simulink model "ControlSingleV1_3"  (R2015b)
settings: Solver=ode1  StartTime=0.0  StopTime=inf  FixedStep=0.001  RelTol=1e-3
libraries: simulink x1
settings Model: ExtModeTrigDuration=10000  Creator=ale  LastModifiedBy=Le
settings SolverCC: PositivePriorityOrder=on
settings RTWCC: SystemTargetFile=quarc_linux_duovero.tlc  TemplateMakefile=quarc_linux_duovero_tmf  Description=QUARC Linux DuoVero Target (QBall 2, QBot 2)
settings STFCustomTargetCC: TargetLibSuffix=.a  TargetPreCompLibLocation=C:\PROGRA~3\QUARC\lib\2015b\LINUX_~1\release  GeneratePreprocessorConditionals=Use local settings  CPPClassGenCompliant=off  SystemTargetFile=quarc_linux_duovero.tlc
settings GRTTargetCC: TargetLibSuffix=.a  TargetPreCompLibLocation=C:\PROGRA~3\QUARC\lib\2015b\LINUX_~1\release  ParMdlRefBuildCompliant=off  CompOptLevelCompliant=off  CombineOutputUpdateFcns=off  MatFileLogging=off  CPPClassGenCompliant=off  GRTInterface=on  UseToolchainInfoCompliant=off  ExtMode=on  ExtModeMexFile=quarc_comm  ExtModeMexArgs='-w -d /tmp -uri %u'

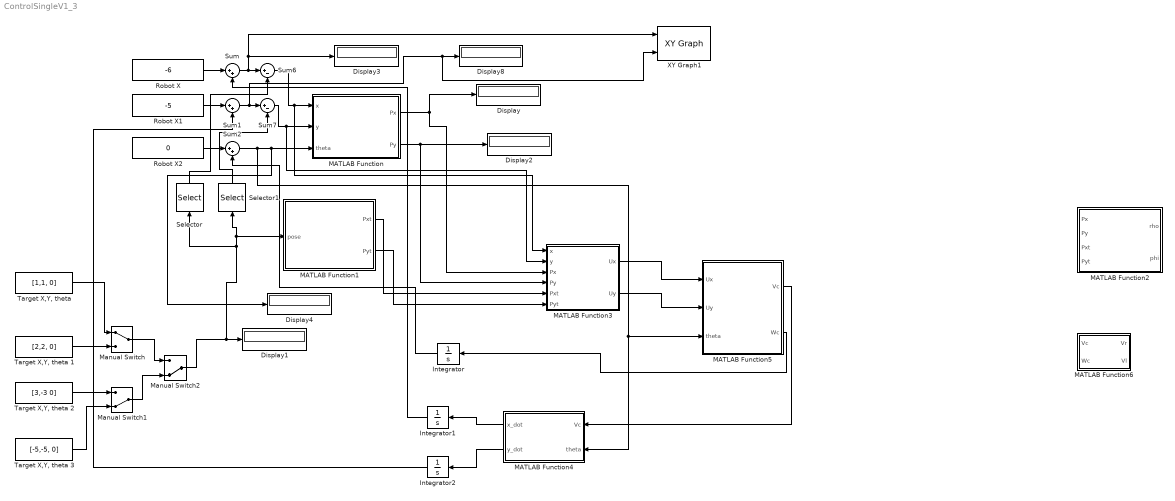
== system ControlSingleV1_3 ==
  Display{,1..4,8} (6 alike) : Display
  Integrator : Integrator
  Integrator1 : Integrator
  Integrator2 : Integrator
  MATLAB Function : MATLAB Function  TreatAsAtomicUnit=on
  MATLAB Function1 : MATLAB Function  TreatAsAtomicUnit=on
  MATLAB Function2 : MATLAB Function  TreatAsAtomicUnit=on
  MATLAB Function3 : MATLAB Function  TreatAsAtomicUnit=on
  MATLAB Function4 : MATLAB Function  TreatAsAtomicUnit=on
  MATLAB Function5 : MATLAB Function  TreatAsAtomicUnit=on
  MATLAB Function6 : MATLAB Function  TreatAsAtomicUnit=on
  Manual Switch : ManualSwitch
  Manual Switch1 : ManualSwitch  CurrentSetting=0
  Manual Switch2 : ManualSwitch  CurrentSetting=0
  Robot X : Constant  Value=-6
  Robot X1 : Constant  Value=-5
  Robot X2 : Constant  Value=0
  Selector : Selector  InputPortWidth=3  IndexOptions=Index vector (dialog)  Indices=[1]  OutputSizes=1
  Selector1 : Selector  InputPortWidth=3  IndexOptions=Index vector (dialog)  Indices=[2]  OutputSizes=1
  Sum : Sum  Inputs=|++
  Sum1 : Sum  Inputs=|++
  Sum2 : Sum  Inputs=|++
  Sum6 : Sum  Inputs=|+-
  Sum7 : Sum  Inputs=|+-
  "Target X,Y, theta " : Constant  Value=[1,1, 0]
  "Target X,Y, theta 1" : Constant  Value=[2,2, 0]
  "Target X,Y, theta 2" : Constant  Value=[3,-3 0]
  "Target X,Y, theta 3" : Constant  Value=[-5,-5, 0]
  XY Graph1 : simulink/Sinks/XY Graph  xmin=-20  xmax=20  ymin=-20  ymax=20  st=-1
  wires:
  MATLAB Function1/1(Pxt) -> MATLAB Function3/5(Pxt)
  MATLAB Function1/2(Pyt) -> MATLAB Function3/6(Pyt)
  MATLAB Function/2(Py) -> MATLAB Function3/4(Py), Display2/1
  MATLAB Function/1(Px) -> MATLAB Function3/3(Px), Display/1
  Sum2/1 -> MATLAB Function4/2(theta), MATLAB Function5/3(theta), Display4/1, MATLAB Function/3(theta)
  Sum7/1 -> MATLAB Function3/2(y), MATLAB Function/2(y)
  Sum6/1 -> MATLAB Function3/1(x), MATLAB Function/1(x)
  Robot X2/1 -> Sum2/1
  Robot X/1 -> Sum/1
  Robot X1/1 -> Sum1/1
  Selector1/1 -> Sum7/2
  Selector/1 -> Sum6/2
  Manual Switch2/1 -> Selector/1, Selector1/1, MATLAB Function1/1(pose), Display1/1
  "Target X,Y, theta "/1 -> Manual Switch/1
  Sum1/1 -> XY Graph1/2, Display8/1, Sum7/1
  Sum/1 -> XY Graph1/1, Display3/1, Sum6/1
  "Target X,Y, theta 1"/1 -> Manual Switch/2
  Manual Switch/1 -> Manual Switch2/1
  Manual Switch1/1 -> Manual Switch2/2
  "Target X,Y, theta 2"/1 -> Manual Switch1/1
  "Target X,Y, theta 3"/1 -> Manual Switch1/2
  MATLAB Function3/1(Ux) -> MATLAB Function5/1(Ux)
  MATLAB Function3/2(Uy) -> MATLAB Function5/2(Uy)
  MATLAB Function5/1(Vc) -> MATLAB Function4/1(Vc)
  MATLAB Function5/2(Wc) -> Integrator/1
  Integrator/1 -> Sum2/2
  MATLAB Function4/1(x_dot) -> Integrator1/1
  Integrator1/1 -> Sum/2
  MATLAB Function4/2(y_dot) -> Integrator2/1
  Integrator2/1 -> Sum1/2

== matlab function ControlSingleV1_3/MATLAB Function1 ==
  data: pose input; Pxt output; Pyt output
function [Pxt,Pyt] = PxtPyt_convert(pose)
x=pose(1);
y=pose(2);
theta=pose(2);
l=.0235; %#length between the two wheels in meters
%R=.0175; %#R or signed distance from ICC (Instanteous center of curvature) in meters
Pxt= x+l*cos(theta)
Pyt = y+l*sin(theta)

%#codegen

== matlab function ControlSingleV1_3/MATLAB Function ==
  data: x input; Px output; Py output; y input; theta input
function [Px,Py] = PxPy_convert(x, y, theta)

l=.0235; %#length between the two wheels in meters
%R=.0175; %#R or signed distance from ICC (Instanteous center of curvature) in meters
Px= x+l*cos(theta)
Py = y+l*sin(theta)

%#codegen

== matlab function ControlSingleV1_3/MATLAB Function2 ==
  data: Px input; rho output; Py input; Pxt input; Pyt input; phi output
function [rho, phi] = rho_phi_convert(Px,Py,Pxt,Pyt)
    [phi, rho] = cart2pol((Px-Pxt),(Py-Pyt))

== matlab function ControlSingleV1_3/MATLAB Function3 ==
  data: x input; y input; Px input; Ux output; Py input; Pxt input; Pyt input; Uy output
function [Ux, Uy] = UxUy(x,y,Px,Py,Pxt,Pyt)
%#codegen
rho_star=.5;
omega_star=.5;
krho = 1
kphi = 1;
w_d=10;
U = [0 0];
rho_size = 1;
phi_size = 1;
[phi, rho] = cart2pol(Px,Py);
[phi_d, rho_d] = cart2pol(Pxt,Pyt);
[phi_dif, rho_dif] = cart2pol((Px-Pxt),(Py-Pyt));

J_i=[x/(sqrt(x^2+y^2)) y/(sqrt(x^2+y^2)); -y/(x^2+y^2) x/(x^2+y^2)];
%J_i=[ (Px-Pxt)/phi (Py-Pyt)/phi;    -(Py-Pyt)/((1+((Py-Pyt)/(Px-Pxt))^2)*(Px-Pxt)^2)  1/((1+((Py-Pyt)/(Px-Pxt))^2)*(Px-Pxt)) ];
%J_i=[ (Px-Pxt)/phi (Py-Pyt)/phi_dif;    -(Py-Pyt)/(phi_dif)^2  (Px-Pxt)/(phi_dif)^2 ];

rhoi_dot = krho*(rho_size-rho)
%phii_d= phi/2
%phii_d = phi_d - phii_d
phii_dot = w_d + kphi*((phi_size-phi)/2);
V_i= [rhoi_dot; phii_dot];
Rt = [ 1 0; 0 1];


U = Rt*(J_i'*V_i);
Ux = U(1);
Uy = U(2);

== matlab function ControlSingleV1_3/MATLAB Function4 ==
  data: Vc input; x_dot output; theta input; y_dot output
function [x_dot, y_dot] = VcWc2XYdot(Vc, theta)
%#codegen
x_dot = Vc*cos(theta)
y_dot = Vc*sin(theta)

== matlab function ControlSingleV1_3/MATLAB Function5 ==
  data: Ux input; Vc output; Uy input; Wc output; theta input
function [Vc,Wc] = UxUy2VcWc(Ux,Uy, theta)

l=.0235; %#length between the two wheels in meters
kin_inv = inv([cos(theta) -l*sin(theta) ; sin(theta) l*cos(theta)]);
P =  kin_inv*[Ux;Uy];
Vc=P(1);
Wc=P(2);

== matlab function ControlSingleV1_3/MATLAB Function6 ==
  data: Vc input; Vr output; Wc input; Vl output
function [Vr,Vl] = VcWc2VrVl(Vc,Wc)
%#codegen

l=.0235;
Vr = Vc+(1/2)*(l*2)*Wc;
Vl = Vc-(1/2)*(l*2)*Wc;
